simulink model "ASML_BaselineController"  (R2020b)
settings: Solver=FixedStepAuto  StartTime=0.0  StopTime=0.02  FixedStep=Ts  RelTol=1e-3
model workspace (MAT data in the model file):
  dUdY = 0.865
  dlgcNominal = 0.5
  iGain = 7500
  intStopTime = 1000
  integratorLimit = inf
  pGain = 0.45
values from neighbouring files (symbols this model uses):
  Ts = 20e-6    (= 2e-05)    [computeDose1Burst.m]    (also in computeDose1Burst_filtered.m; modelParams.mat)
undefined symbols (not defined in the file or in its folder): DiscIntNeverNeededParam
libraries: simulink x2
settings Model: OrderedModelArguments=off  Creator=rjacques  LastModifiedBy=andliu
settings DataIOCC: ExternalInput=extInput_Rfcm2ShotsBehind  DSMLogging=off  SaveTime=off  ReturnWorkspaceOutputs=off
settings DebuggingCC: ArithmeticOperatorsInVariantConditions=warning
settings SFSimCC: CustomCodeUndefinedFunction=UseInterfaceOnly
settings GRTTargetCC: CombineOutputUpdateFcns=off  MatFileLogging=off

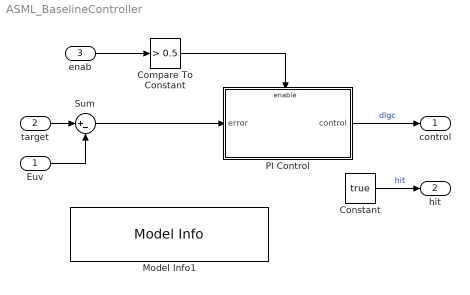
== system ASML_BaselineController ==
  "Euv " : Inport
  target : Inport  Port=2
  enab : Inport  Port=3
  Compare To Constant : simulink/Logic and Bit Operations/Compare To Constant  relop=>  const=0.5  OutDataTypeStr=boolean
  Constant : Constant  Value=true
  Model Info1 : simulink/Model-Wide Utilities/Model Info  Frame=on  DisplayStringWithTags=|  HorizontalTextAlignment=Left  LeftAlignmentValue=0.02
      | %<ModelName>
      | Simulink model version: %<ModelVersion>
      | Modified on: %<LastModificationDate>
      | Modified by: %<ModifiedBy>
  PI Control : Subsystem
  Sum : Sum  Inputs=|+-
  control : Outport  VectorParamsAs1DForOutWhenUnconnected=off
  hit : Outport  Port=2  VectorParamsAs1DForOutWhenUnconnected=off
  wires:
  target/1 -> Sum/1
  Sum/1 -> PI Control/1(error)
  "Euv "/1 -> Sum/2
  enab/1 -> Compare To Constant/1
  PI Control/1(control) -> control/1  "dlgc"
  Constant/1 -> hit/1  "hit"
  Compare To Constant/1 -> PI Control/Enable

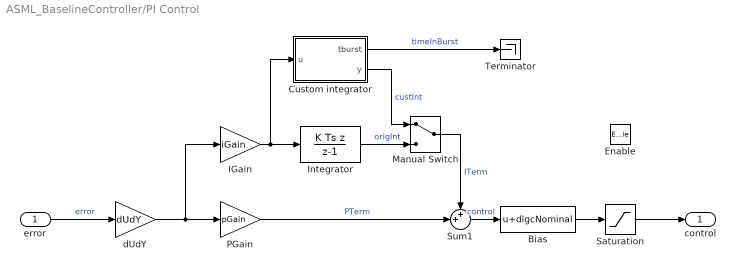
== system ASML_BaselineController/PI Control ==
  error : Inport
  Enable : EnablePort  StatesWhenEnabling=reset
  Bias : Bias  Bias=dlgcNominal
  Custom integrator : Subsystem
  IGain : Gain  Gain=iGain
  Integrator : DiscreteIntegrator  IntegratorMethod=Integration: Backward Euler  gainval=1  InitialCondition=min(0,integratorLimit)  SampleTime=-1  LimitOutput=on  UpperSaturationLimit=integratorLimit  ICPrevOutput=DiscIntNeverNeededParam  ICPrevScaledInput=DiscIntNeverNeededParam
  Manual Switch : ManualSwitch
  PGain : Gain  Gain=pGain
  Saturation : Saturate  UpperLimit=1  LowerLimit=-inf
  Sum1 : Sum  Inputs=++|
  Terminator : Terminator
  dUdY : Gain  Gain=dUdY
  control : Outport  OutputWhenDisabled=reset  InitialOutput=dlgcNominal  VectorParamsAs1DForOutWhenUnconnected=off
  wires:
  Bias/1 -> Saturation/1
  error/1 -> dUdY/1  "error"
  Sum1/1 -> Bias/1  "control"
  IGain/1 -> Custom integrator/1(u), Integrator/1
  Integrator/1 -> Manual Switch/2  "origInt"
  PGain/1 -> Sum1/2  "PTerm"
  dUdY/1 -> IGain/1, PGain/1
  Saturation/1 -> control/1
  Custom integrator/1(tburst) -> Terminator/1  "timeInBurst"
  Custom integrator/2(y) -> Manual Switch/1  "custInt"
  Manual Switch/1 -> Sum1/1  "ITerm"

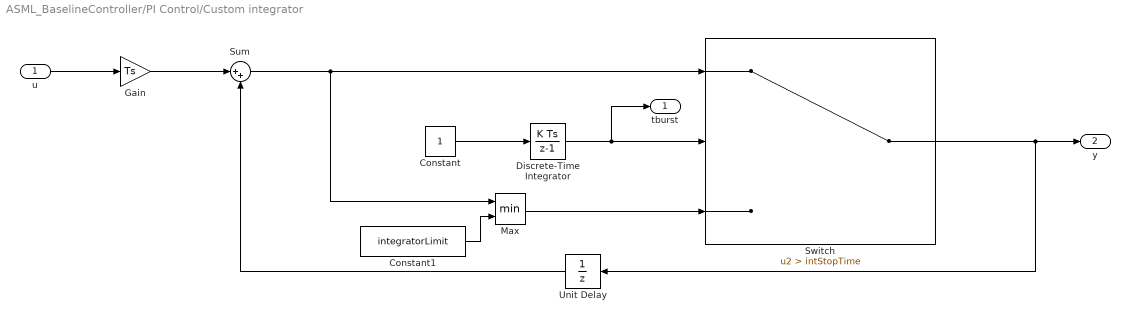
== system ASML_BaselineController/PI Control/Custom integrator ==
  u : Inport
  Constant : Constant
  Constant1 : Constant  Value=integratorLimit
  Discrete-Time Integrator : DiscreteIntegrator  gainval=1  SampleTime=-1  ICPrevOutput=DiscIntNeverNeededParam  ICPrevScaledInput=DiscIntNeverNeededParam
  Gain : Gain  Gain=Ts
  Max : MinMax  Inputs=2
  Sum : Sum  Inputs=|++
  Switch : Switch  Criteria=u2 > Threshold  Threshold=intStopTime
  Unit Delay : UnitDelay  SampleTime=-1  HasFrameUpgradeWarning=on
  tburst : Outport
  y : Outport  Port=2
  wires:
  u/1 -> Gain/1
  Discrete-Time Integrator/1 -> tburst/1, Switch/2
  Constant/1 -> Discrete-Time Integrator/1
  Sum/1 -> Max/1, Switch/1
  Unit Delay/1 -> Sum/2
  Gain/1 -> Sum/1
  Constant1/1 -> Max/2
  Max/1 -> Switch/3
  Switch/1 -> Unit Delay/1, y/1
